simulink model "temp_acc_ext_test"  (R2024a)
settings: Solver=VariableStepAuto  StartTime=0.0  StopTime=0.2  RelTol=1e-3
undefined symbols (not defined in the file): B_para, L_t, mmp_fir_coeff, mmp_iir_coeff, T_cs, T_fs, T_ss, w_d
settings Model: Creator=tpjch  LastModifiedBy=tpjch

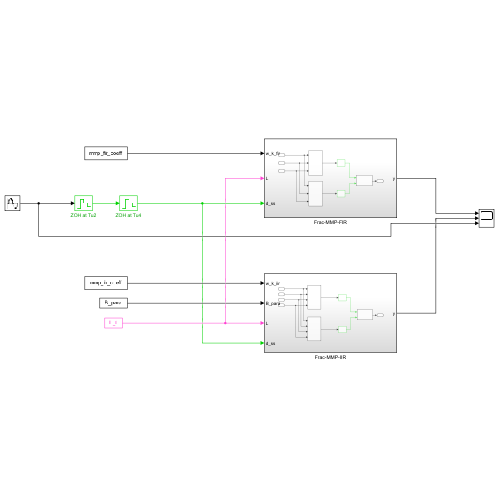
[thumbnail: Simulink's stored preview of the top-level diagram]
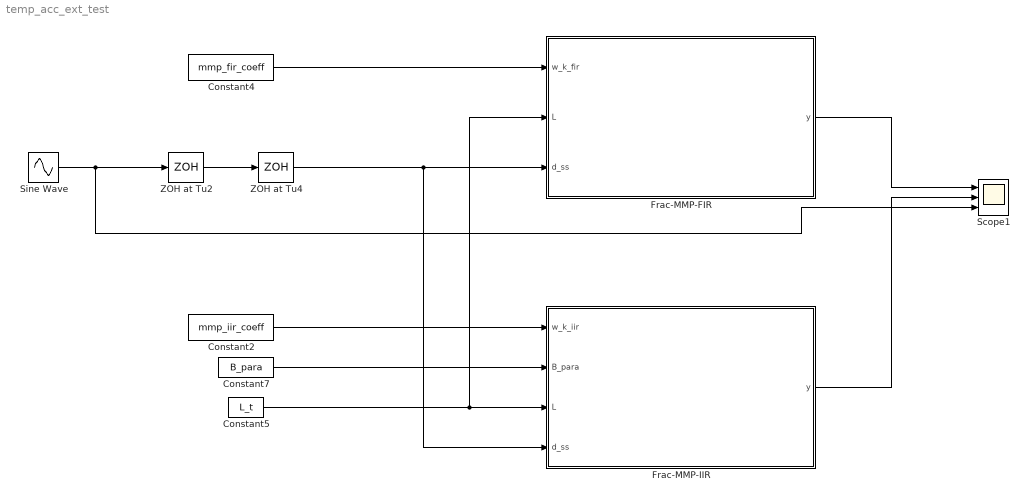
== system temp_acc_ext_test ==
  Constant2 : Constant  Value=mmp_iir_coeff
  Constant4 : Constant  Value=mmp_fir_coeff
  Constant5 : Constant  Value=L_t
  Constant7 : Constant  Value=B_para
  Frac-MMP-FIR : Subsystem
  Frac-MMP-IIR : Subsystem
  Scope1 : Scope  NumInputPorts=3
  Sine Wave : Sin  Frequency=w_d/T_fs  SampleTime=T_cs/50
  ZOH at Tu2 : ZeroOrderHold  SampleTime=T_ss
  ZOH at Tu4 : ZeroOrderHold  SampleTime=T_cs
  wires:
  ZOH at Tu2/1 -> ZOH at Tu4/1
  Frac-MMP-IIR/1(y) -> Scope1/2
  Constant2/1 -> Frac-MMP-IIR/1(w_k_iir)
  Constant7/1 -> Frac-MMP-IIR/2(B_para)
  Frac-MMP-FIR/1(y) -> Scope1/1
  Constant4/1 -> Frac-MMP-FIR/1(w_k_fir)
  Constant5/1 -> Frac-MMP-FIR/2(L), Frac-MMP-IIR/3(L)
  ZOH at Tu4/1 -> Frac-MMP-IIR/4(d_ss), Frac-MMP-FIR/3(d_ss)
  Sine Wave/1 -> Scope1/3, ZOH at Tu2/1

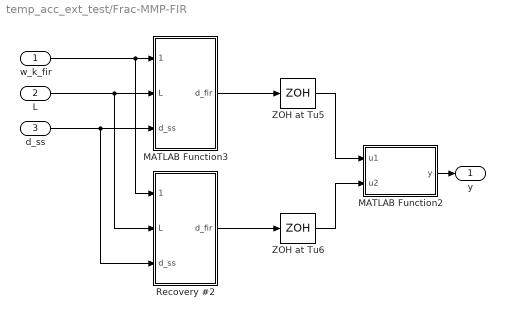
== system temp_acc_ext_test/Frac-MMP-FIR ==
  w_k_fir : Inport
  L : Inport  Port=2
  d_ss : Inport  Port=3
  MATLAB Function2 : MATLAB Function  TreatAsAtomicUnit=on
  MATLAB Function3 : MATLAB Function  TreatAsAtomicUnit=on  SystemSampleTime=T_cs
  Recovery #2 : MATLAB Function  TreatAsAtomicUnit=on  SystemSampleTime=T_cs
  ZOH at Tu5 : ZeroOrderHold  SampleTime=T_cs
  ZOH at Tu6 : ZeroOrderHold  SampleTime=T_cs
  y : Outport
  wires:
  MATLAB Function2/1(y) -> y/1
  L/1 -> Recovery #2/2(L), MATLAB Function3/2(L)
  w_k_fir/1 -> Recovery #2/1(w_k_fir), MATLAB Function3/1(w_k_fir)
  ZOH at Tu5/1 -> MATLAB Function2/1(u1)
  MATLAB Function3/1(d_fir) -> ZOH at Tu5/1
  Recovery #2/1(d_fir) -> ZOH at Tu6/1
  ZOH at Tu6/1 -> MATLAB Function2/2(u2)
  d_ss/1 -> Recovery #2/3(d_ss), MATLAB Function3/3(d_ss)

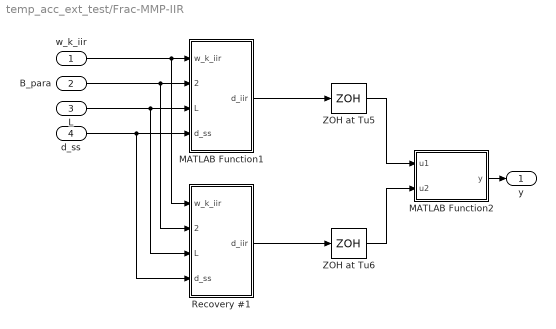
== system temp_acc_ext_test/Frac-MMP-IIR ==
  w_k_iir : Inport
  B_para : Inport  Port=2
  L : Inport  Port=3
  d_ss : Inport  Port=4
  MATLAB Function1 : MATLAB Function  TreatAsAtomicUnit=on  SystemSampleTime=T_cs
  MATLAB Function2 : MATLAB Function  TreatAsAtomicUnit=on
  Recovery #1 : MATLAB Function  TreatAsAtomicUnit=on  SystemSampleTime=T_cs
  ZOH at Tu5 : ZeroOrderHold  SampleTime=T_cs
  ZOH at Tu6 : ZeroOrderHold  SampleTime=T_cs
  y : Outport
  wires:
  MATLAB Function2/1(y) -> y/1
  L/1 -> Recovery #1/3(L), MATLAB Function1/3(L)
  w_k_iir/1 -> Recovery #1/1(w_k_iir), MATLAB Function1/1(w_k_iir)
  ZOH at Tu5/1 -> MATLAB Function2/1(u1)
  MATLAB Function1/1(d_iir) -> ZOH at Tu5/1
  Recovery #1/1(d_iir) -> ZOH at Tu6/1
  ZOH at Tu6/1 -> MATLAB Function2/2(u2)
  B_para/1 -> Recovery #1/2(B_para), MATLAB Function1/2(B_para)
  d_ss/1 -> Recovery #1/4(d_ss), MATLAB Function1/4(d_ss)

== matlab function temp_acc_ext_test/Frac-MMP-IIR/Recovery #1 ==
  settings: updateMethod=DISCRETE
  data: w_k_iir input; B_para input; L input; d_ss input; d_iir output
function d_iir  = fcn(w_k_iir, B_para, L, d_ss)
    % Keeps data of variables
    persistent  n_w phi n_cs n_ss d_buff d_fs_iir max_buffer_size buffer_indices N_L D_L
    % Assigning initial values   
    if isempty(n_w)
        n_w = size(w_k_iir,1); % n_w = 2m disturbances (index starts at 0,1,...,2m-1)
        phi = zeros(1, n_w, 'like', d_ss); % Preallocate phi using the same type as d_ss
        [N_L, D_L] = rat(L);
        n_cs = -N_L; % offset to be one slow sample behind, rate at T_fs/D_L
        n_ss = 0; % Slow sampling count
        d_fs_iir = 0;
        buffer_indices = 2:N_L:((n_w-1) * N_L + 2);
        max_buffer_size = (n_w * N_L + 1);
        d_buff = zeros(1, max_buffer_size, 'like', d_ss);
    end
    
    % Increment fast sampling count
    n_cs = n_cs + 1;
    k = mod(n_cs-1,2*N_L); % check if on intersample
    % Update slow sampling count when k == 0
    if k == 0
        n_ss = n_ss + 1; % Number of slow samples
    end

    % Case 1: n_ss < n_w (not enough data points for FIR)
    if n_ss < n_w
        if k == 0 % Fast and slow align
            phi = [d_ss, phi(1:end-1)]; % Shift and update phi
            d_iir = d_ss;
            d_buff = [d_iir, d_buff(1:end-1)];
        else % Not enough data for intersample estimation
            d_iir = 0;
            d_buff = [d_iir, d_buff(1:end-1)];
        end
    % Case 2: n_ss >= n_w (enough data points for FIR)
    elseif n_ss >= n_w && n_ss < (n_w + 1)
        if k == 0 
            phi = [d_ss, phi(1:end-1)];
            d_iir = d_ss;
            d_buff = [d_iir, d_buff(1:end-1)];
        elseif k ~= 0 && mod(k,2) == 0 % FIR reconstruction
            d_iir = 0;
            d_buff = [d_iir, d_buff(1:end-1)];
        else k ~= 0 && mod(k+1,2) == 0;
            d_iir = 0;
        end
    % Case 3: n_w >= n_w+1, IIR reconstruction
    else
        if k == 0
            phi = [d_ss, phi(1:end-1)];
            d_iir = d_ss;
            d_buff = [d_iir, d_buff(1:end-1)];
        elseif k ~= 0 && mod(k,2) == 0
            d_temp = flip(d_buff);
            d_iir = phi * w_k_iir(:,k/D_L) - ...
                    d_temp(buffer_indices) * flip(B_para(2:end));
            d_buff = [d_iir, d_buff(1:end-1)];
        else k ~= 0 && mod(k+1,2) == 0;
            d_iir = d_fs_iir;
        end
    end
end

== matlab function temp_acc_ext_test/Frac-MMP-IIR/MATLAB Function1 ==
  settings: updateMethod=DISCRETE
  data: w_k_iir input; B_para input; L input; d_ss input; d_iir output
function d_iir  = fcn(w_k_iir, B_para, L, d_ss)
    % Keeps data of variables
    persistent  n_w phi n_cs n_ss d_buff d_fs_iir max_buffer_size buffer_indices N_L D_L
    % Assigning initial values   
    if isempty(n_w)
        n_w = size(w_k_iir,1); % n_w = 2m disturbances (index starts at 0,1,...,2m-1)
        phi = zeros(1, n_w, 'like', d_ss); % Preallocate phi using the same type as d_ss
        n_cs = 0; % combined sampling count, rate at T_fs/N_L
        n_ss = 0; % Slow sampling count
        d_fs_iir = 0;
        [N_L, D_L] = rat(L);
        buffer_indices = 2:N_L:((n_w-1) * N_L + 2);
        max_buffer_size = (n_w * N_L + 1);
        d_buff = zeros(1, max_buffer_size, 'like', d_ss);
    end
    
    % Increment fast sampling count
    n_cs = n_cs + 1;
    k = mod(n_cs-1,2*N_L); % check if on intersample
    % Update slow sampling count when k == 0
    if k == 0
        n_ss = n_ss + 1; % Number of slow samples
    end

    % Case 1: n_ss < n_w (not enough data points for FIR)
    if n_ss < n_w
        if k == 0 % Fast and slow align
            phi = [d_ss, phi(1:end-1)]; % Shift and update phi
            d_iir = d_ss;
            d_buff = [d_iir, d_buff(1:end-1)];
        else % Not enough data for intersample estimation
            d_iir = 0;
            d_buff = [d_iir, d_buff(1:end-1)];
        end
    % Case 2: n_ss >= n_w (enough data points for FIR)
    elseif n_ss >= n_w && n_ss < (n_w + 1)
        if k == 0 
            phi = [d_ss, phi(1:end-1)];
            d_iir = d_ss;
            d_buff = [d_iir, d_buff(1:end-1)];
        elseif k ~= 0 && mod(k,2) == 0 % FIR reconstruction
            d_iir = 0;
            d_buff = [d_iir, d_buff(1:end-1)];
        else k ~= 0 && mod(k+1,2) == 0;
            d_iir = 0;
        end
    % Case 3: n_w >= n_w+1, IIR reconstruction
    else
        if k == 0
            phi = [d_ss, phi(1:end-1)];
            d_iir = d_ss;
            d_buff = [d_iir, d_buff(1:end-1)];
        elseif k ~= 0 && mod(k,2) == 0
            d_temp = flip(d_buff);
            d_iir = phi * w_k_iir(:,k/D_L) - ...
                    d_temp(buffer_indices) * flip(B_para(2:end));
            d_fs_iir = d_iir;
            d_buff = [d_iir, d_buff(1:end-1)];
        else k ~= 0 && mod(k+1,2) == 0;
            d_iir = d_fs_iir;
        end
    end
    % update buffer
end

== matlab function temp_acc_ext_test/Frac-MMP-IIR/MATLAB Function2 ==
  data: u1 input; y output; u2 input
function y = summation(u1,u2)

persistent k

if isempty(k)
    k = uint32(0);
end

if mod(k,2) == 0
    y = u1;
else
    y = u2;
end

k = k + 1;

== matlab function temp_acc_ext_test/Frac-MMP-FIR/MATLAB Function2 ==
  data: u1 input; y output; u2 input
function y = summation(u1,u2)

persistent k

if isempty(k)
    k = uint32(0);
end

if mod(k,2) == 0
    y = u1;
else
    y = u2;
end

k = k + 1;

== matlab function temp_acc_ext_test/Frac-MMP-FIR/MATLAB Function3 ==
  settings: updateMethod=DISCRETE
  data: w_k_fir input; L input; d_ss input; d_fir output size=1
function d_fir  = fcn(w_k_fir, L, d_ss)
    % Keeps data of variables
    persistent  n_w phi n_cs n_ss d_fs_fir D_L N_L
    % Assigning initial values   
    if isempty(n_w)
        n_w = size(w_k_fir,1); % n_w = 2m disturbances (index starts at 0,1,...,2m-1)
        phi = zeros(1, n_w, 'like', d_ss); % Preallocate phi using the same type as d_ss
        n_cs = 0; % combined sampling count, rate at T_fs/N_L
        n_ss = 0; % Slow sampling count
        d_fs_fir = 0; % store previous value for the estimate
        [N_L, D_L] = rat(L);
    end
    
    % Increment fast sampling count
    n_cs = n_cs + 1;
    k = mod(n_cs-1,2*N_L); % check if on intersample
    % Update slow sampling count when k == 0
    if k == 0
        n_ss = n_ss + 1; % Number of slow samples
    end

    % Case 1: n_ss < n_w (not enough data points for FIR)
    if n_ss < n_w
        if k == 0 % Fast and slow align
            phi = [d_ss, phi(1:end-1)]; % Shift and update phi
            d_fir = d_ss;
        else % Not enough data for intersample estimation
            d_fir = 0;
        end
    % Case 2: n_ss >= n_w (enough data points for FIR)
    else
        if k == 0 
            phi = [d_ss, phi(1:end-1)];
            d_fir = d_ss;
        elseif k ~= 0 && mod(k,2) == 0 % FIR reconstruction
            d_fir = phi * w_k_fir(:, k/D_L); 
            d_fs_fir = d_fir;
        else k ~= 0 && mod(k+1,2) == 0;
            d_fir = d_fs_fir;
        end
    % update buffer
    end

== matlab function temp_acc_ext_test/Frac-MMP-FIR/Recovery #2 ==
  settings: updateMethod=DISCRETE
  data: w_k_fir input; L input; d_ss input; d_fir output size=1
function d_fir = fcn(w_k_fir, L, d_ss)
    % Keeps data of variables
    persistent  n_w phi n_cs n_ss d_fs_fir N_L D_L
    % Assigning initial values   
    if isempty(n_w)
        n_w = size(w_k_fir,1); % n_w = 2m disturbances (index starts at 0,1,...,2m-1)
        phi = zeros(1, n_w, 'like', d_ss); % Preallocate phi using the same type as d_ss
        [N_L, D_L] = rat(L);
        n_cs = -N_L; % offset to be one slow sample behind, rate at T_fs/D_L
        n_ss = 0; % Slow sampling count
        d_fs_fir = 0; % store previous value for the estimate
    end
    
    % Increment fast sampling count
    n_cs = n_cs + 1;
    k = mod(n_cs-1,2*N_L); % check if on intersample
    % Update slow sampling count when k == 0
    if k == 0
        n_ss = n_ss + 1; % Number of slow samples
    end

    % Case 1: n_ss < n_w (not enough data points for FIR)
    if n_ss < n_w
        if k == 0 % Fast and slow align
            phi = [d_ss, phi(1:end-1)]; % Shift and update phi
            d_fir = d_ss;
        else % Not enough data for intersample estimation
            d_fir = 0;
        end
    % Case 2: n_ss >= n_w (enough data points for FIR)
    else
        if k == 0 
            phi = [d_ss, phi(1:end-1)];
            d_fir = d_ss;
        elseif k ~= 0 && mod(k,2) == 0 % FIR reconstruction
            d_fir = phi * w_k_fir(:, k/D_L); 
            d_fs_fir = d_fir;
        else k ~= 0 && mod(k+1,2) == 0;
            d_fir = d_fs_fir;
        end
    end
